simulink model "overall_model"  (R2025b)
settings: Solver=VariableStepAuto  StartTime=0.0  StopTime=10.0  RelTol=1e-3
values from neighbouring files (symbols this model uses):
  mu = 3.986004418e14    (= 398600441800000)    [initialize_orbital_dynamics.m]
  r0 = [r0_mag; 0; 0]    [initialize_orbital_dynamics.m]
  v0 = [0; v0_mag; 0]    [initialize_orbital_dynamics.m]
undefined symbols (not defined in the file or in its folder): A, I, N, WMM2020
libraries: aerolibtransform2 x1, aerolibgravity2 x1, sharedutil x1, matrix_library x1
settings Model: Creator=jennaparker  LastModifiedBy=mahausmani

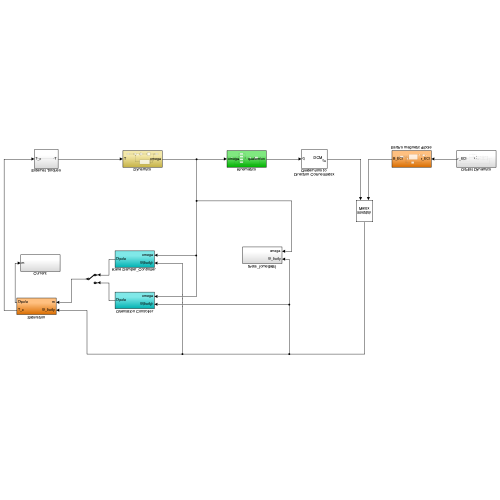
[thumbnail: Simulink's stored preview of the top-level diagram]
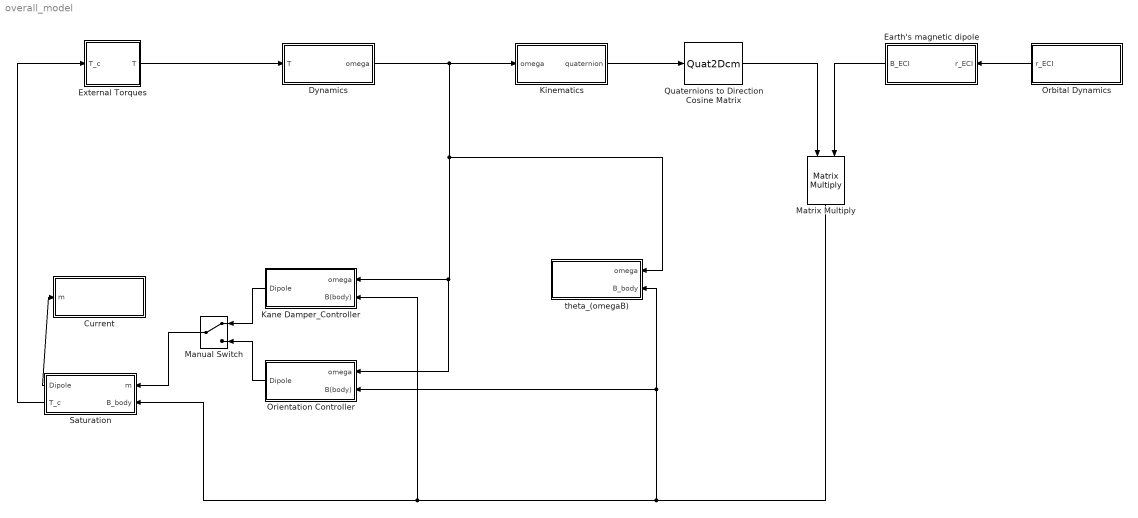
== system overall_model ==
  Current : Subsystem
  Dynamics : Subsystem
  Earth's magnetic dipole : Subsystem
  External Torques : Subsystem
  "Kane Damper_Controller " : Subsystem
  Kinematics : Subsystem
  Manual Switch : ManualSwitch
  Matrix Multiply : Product  Multiplication=Matrix(*)
  Orbital Dynamics : Subsystem
  Orientation Controller : Subsystem
  Quaternions to Direction Cosine Matrix : Quat2Dcm
  Saturation : Subsystem
  theta_(omegaB) : Subsystem
  wires:
  Orbital Dynamics/1(r_ECI) -> Earth's magnetic dipole/1(r_ECI)
  Earth's magnetic dipole/1(B_ECI) -> Matrix Multiply/2
  Quaternions to Direction Cosine Matrix/1 -> Matrix Multiply/1
  Kinematics/1(quaternion) -> Quaternions to Direction Cosine Matrix/1
  Dynamics/1(omega) -> Kinematics/1(omega), Orientation Controller/1(omega), "Kane Damper_Controller "/1(omega), theta_(omegaB)/1(omega)
  Saturation/1(Dipole) -> Current/1("m ")
  Saturation/2(T_c) -> External Torques/1(T_c)
  "Kane Damper_Controller "/1(Dipole) -> Manual Switch/1
  Orientation Controller/1(Dipole) -> Manual Switch/2
  Manual Switch/1 -> Saturation/1(m)
  Matrix Multiply/1 -> Orientation Controller/2(B(body)), theta_(omegaB)/2(B_body), Saturation/2(B_body), "Kane Damper_Controller "/2(B(body))
  External Torques/1(T) -> Dynamics/1(T)

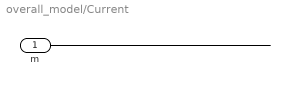
== system overall_model/Current ==
  "m " : Inport
  wires:
  "m "/1 -> ?

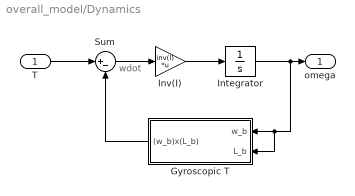
== system overall_model/Dynamics ==
  note: wdot
  T : Inport
  Gyroscopic T : Subsystem
      settings: PortSchema="{\"entries\":[{\"content\":{\"sides\":[{\"content\":{\"connectorIds\":[\"Out1\"]},\"type\":\"ConnectorPlacement.EquallySpacedRectSide\",\"uuid\":\"212ee7dd-a66b-44a5-ab1b-fc35ef6a11df\"},{\"content\":{\"connectorIds\":[\"In1\",\"In2\"],\"side\":\"RIGHT\"},\"type\":\"ConnectorPlacement.EquallySpacedRectSide\",\"uuid\":\"a8c03a11-e631-42c9-9641-96e88dbd14f3\"},{\"content\":{\"side\":\"TOP\"},\"type\":\"ConnectorPlacement.EquallySpacedRectSide\",\"uuid\":\"084a92ad-2c56-4bcb-add2-55144b69ebb8\"},{\"content\":{\"side\":\"BOTTOM\"},\"type\":\"ConnectorPlacement.EquallySpacedRectSide\",\"uuid\":\"daa02227-9ed0-4aaf-8c4f-a961aaf032a5\"}]},\"type\":\"ConnectorPlacement.EquallySpacedConnector\",\"uuid\":\"efdd6a42-0687-403c-ac74-0775edd64043\"}],\"packageUris\":[\"http://schema.mathworks.com/mf0/Connector/R2020b\"],\"version\":\"1.0\"}"
  Integrator : Integrator
  Inv(I) : Gain  Gain=inv(I)  Multiplication=Matrix(K*u)
  Sum : Sum  Inputs=|+-
  omega : Outport
  wires:
  Inv(I)/1 -> Integrator/1
  Integrator/1 -> omega/1, Gyroscopic T/2(L_b), Gyroscopic T/1(w_b)
  T/1 -> Sum/1
  Gyroscopic T/1((w_b)x(L_b)) -> Sum/2
  Sum/1 -> Inv(I)/1

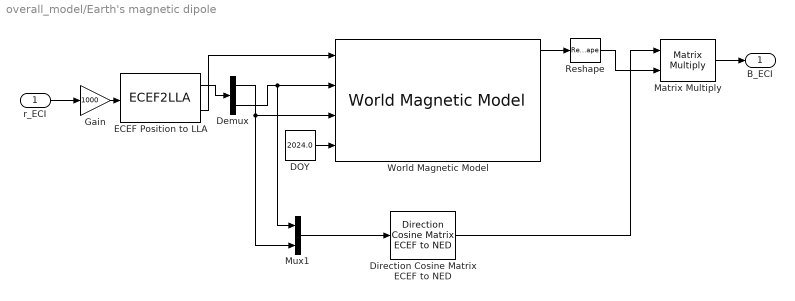
== system overall_model/Earth's magnetic dipole ==
  r_ECI : Inport
  DOY : Constant  Value=2024.0
  Demux : Demux  Outputs=2
  Direction Cosine Matrix ECEF to NED : aerolibtransform2/Direction Cosine Matrix ECEF to NED
  ECEF Position to LLA : ECEF2LLA
  Gain : Gain  Gain=1000
  Matrix Multiply : Product  Multiplication=Matrix(*)
  Mux1 : Mux  Inputs=2
  Reshape : Reshape  OutputDimensionality=Column vector (2-D)
  World Magnetic Model : aerolibgravity2/World Magnetic Model  model=WMM2020 (2020-2025)  customFile='WMM2020.COF'  units=Metric (MKS)  time_in=on  month=January  day=1  year=2020  action=Error  h_out=on  dec_out=on  inc_out=on  ti_out=on
  B_ECI : Outport
  wires:
  Demux/2 -> Mux1/1, World Magnetic Model/2
  Direction Cosine Matrix ECEF to NED/1 -> Matrix Multiply/1
  ECEF Position to LLA/2 -> World Magnetic Model/1
  Matrix Multiply/1 -> B_ECI/1
  World Magnetic Model/1 -> Reshape/1
  Demux/1 -> Mux1/2, World Magnetic Model/3
  DOY/1 -> World Magnetic Model/4
  Mux1/1 -> Direction Cosine Matrix ECEF to NED/1
  ECEF Position to LLA/1 -> Demux/1
  r_ECI/1 -> Gain/1
  Reshape/1 -> Matrix Multiply/2
  Gain/1 -> ECEF Position to LLA/1

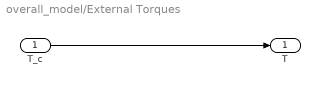
== system overall_model/External Torques ==
  T_c : Inport
  T : Outport
  wires:
  T_c/1 -> T/1

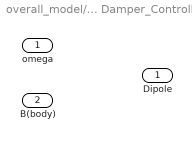
== system overall_model/Kane Damper_Controller  ==
  omega : Inport
  B(body) : Inport  Port=2
  Dipole : Outport

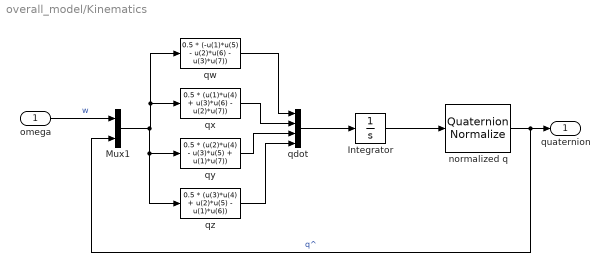
== system overall_model/Kinematics ==
  omega : Inport
  Integrator : Integrator
  Mux1 : Mux  Inputs=2
  normalized q : sharedutil/Quaternion Normalize  aMode=aMode
  qdot : Mux
  qw : Fcn  Expr=0.5 * (-u(1)*u(5) - u(2)*u(6) - u(3)*u(7))
  qx : Fcn  Expr=0.5 * (u(1)*u(4) + u(3)*u(6) - u(2)*u(7))
  qy : Fcn  Expr=0.5 * (u(2)*u(4) - u(3)*u(5) + u(1)*u(7))
  qz : Fcn  Expr=0.5 * (u(3)*u(4) + u(2)*u(5) - u(1)*u(6))
  quaternion : Outport
  wires:
  qz/1 -> qdot/4
  normalized q/1 -> quaternion/1, Mux1/2  "q^"
  qdot/1 -> Integrator/1
  omega/1 -> Mux1/1  "w"
  qy/1 -> qdot/3
  Mux1/1 -> qz/1, qy/1, qx/1, qw/1
  Integrator/1 -> normalized q/1
  qw/1 -> qdot/1
  qx/1 -> qdot/2

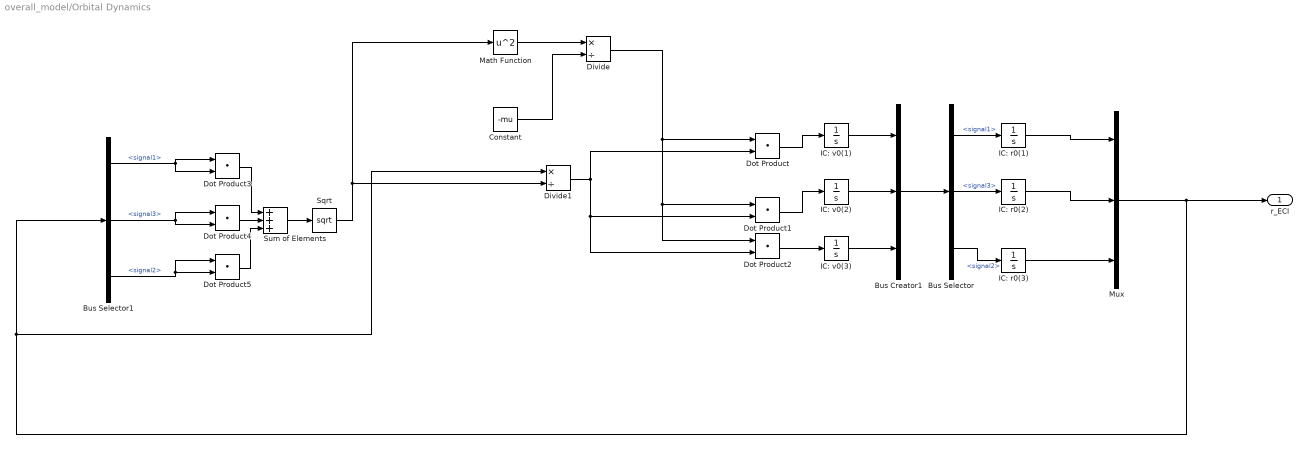
== system overall_model/Orbital Dynamics ==
  Bus Creator1 : BusCreator  Inputs=3
  Bus Selector : BusSelector  OutputSignals=signal1,signal3,signal2
  Bus Selector1 : BusSelector  OutputSignals=signal1,signal3,signal2
  Constant : Constant  Value=-mu
  Divide : Product  Inputs=*/
  Divide1 : Product  Inputs=*/
  Dot Product{,1..5} (6 alike) : DotProduct  OutDataTypeStr=Inherit: Inherit via internal rule
  IC: r0(1) : Integrator  InitialCondition=r0(1)
  IC: r0(2) : Integrator  InitialCondition=r0(2)
  IC: r0(3) : Integrator  InitialCondition=r0(3)
  IC: v0(1) : Integrator  InitialCondition=v0(1)
  IC: v0(2) : Integrator  InitialCondition=v0(2)
  IC: v0(3) : Integrator  InitialCondition=v0(3)
  Math Function : Math  Operator=square
  Mux : Mux  Inputs=3
  Sqrt : Sqrt
  Sum of Elements : Sum  Inputs=+++
  r_ECI : Outport
  wires:
  Bus Selector1/2 -> Dot Product4/1, Dot Product4/2  "<signal3>"
  Divide/1 -> Dot Product2/1, Dot Product1/1, Dot Product/1
  IC: v0(1)/1 -> Bus Creator1/1
  Bus Selector/2 -> IC: r0(2)/1  "<signal3>"
  Sum of Elements/1 -> Sqrt/1
  Dot Product/1 -> IC: v0(1)/1
  Dot Product3/1 -> Sum of Elements/1
  Bus Selector/1 -> IC: r0(1)/1  "<signal1>"
  IC: v0(3)/1 -> Bus Creator1/3
  IC: v0(2)/1 -> Bus Creator1/2
  Bus Selector1/3 -> Dot Product5/1, Dot Product5/2  "<signal2>"
  Math Function/1 -> Divide/1
  Dot Product4/1 -> Sum of Elements/2
  IC: r0(3)/1 -> Mux/3
  Mux/1 -> r_ECI/1, Divide1/1, Bus Selector1/1
  Dot Product2/1 -> IC: v0(3)/1
  Dot Product5/1 -> Sum of Elements/3
  Sqrt/1 -> Divide1/2, Math Function/1
  Bus Creator1/1 -> Bus Selector/1
  Divide1/1 -> Dot Product2/2, Dot Product1/2, Dot Product/2
  Bus Selector1/1 -> Dot Product3/2, Dot Product3/1  "<signal1>"
  Bus Selector/3 -> IC: r0(3)/1  "<signal2>"
  Dot Product1/1 -> IC: v0(2)/1
  Constant/1 -> Divide/2
  IC: r0(1)/1 -> Mux/1
  IC: r0(2)/1 -> Mux/2

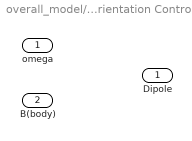
== system overall_model/Orientation Controller ==
  omega : Inport
  B(body) : Inport  Port=2
  Dipole : Outport

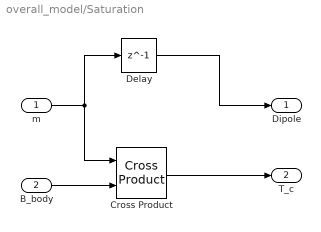
== system overall_model/Saturation ==
  m : Inport
  B_body : Inport  Port=2
  Cross Product : matrix_library/Cross Product
  Delay : Delay  DelayLength=1  InitialCondition=0  SampleTime=1/N*A
  Dipole : Outport
  T_c : Outport  Port=2
  wires:
  m/1 -> Cross Product/1, Delay/1
  B_body/1 -> Cross Product/2
  Cross Product/1 -> T_c/1
  Delay/1 -> Dipole/1

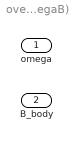
== system overall_model/theta_(omegaB) ==
  omega : Inport
  B_body : Inport  Port=2

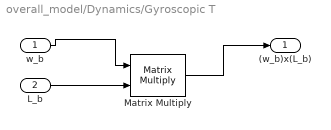
== system overall_model/Dynamics/Gyroscopic T ==
  w_b : Inport
  L_b : Inport  Port=2
  Matrix Multiply : Product  Multiplication=Matrix(*)
  (w_b)x(L_b) : Outport
  wires:
  w_b/1 -> Matrix Multiply/1
  L_b/1 -> Matrix Multiply/2
  Matrix Multiply/1 -> (w_b)x(L_b)/1
